simulink model "tumbling_sim_v4"  (R2018a)
settings: Solver=VariableStepAuto  StartTime=0.0  StopTime=10
values from neighbouring files (symbols this model uses):
  q0 = [0.8034 0.1600 0.4272 0.3828]'    [init_tumbling.m]
  qd0 = [0.0379 0.6999 -0.2503 -0.0927]'    [init_tumbling.m]
settings Model: Creator=abinalexpothen  LastModifiedBy=abinalexpothen

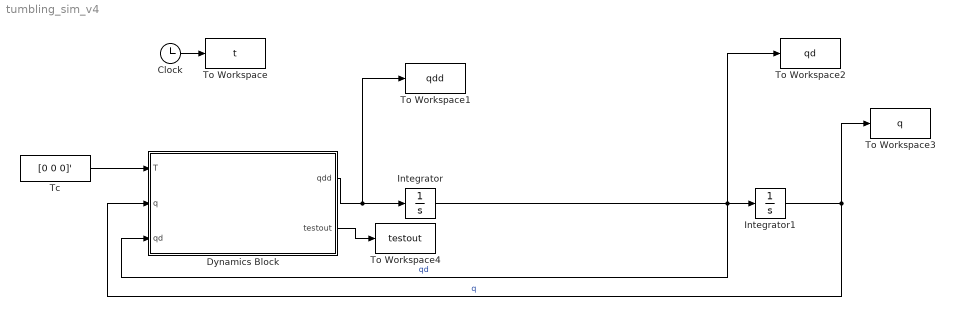
== system tumbling_sim_v4 ==
  Clock : Clock
  Dynamics Block : MATLAB Function  TreatAsAtomicUnit=on
  Integrator : Integrator  InitialCondition=qd0
  Integrator1 : Integrator  InitialCondition=q0
  Tc : Constant  Value=[0 0 0]'
  To Workspace : ToWorkspace  VariableName=t  SampleTime=-1
  To Workspace1 : ToWorkspace  VariableName=qdd  SampleTime=-1
  To Workspace2 : ToWorkspace  VariableName=qd  SampleTime=-1
  To Workspace3 : ToWorkspace  VariableName=q  SampleTime=-1
  To Workspace4 : ToWorkspace  VariableName=testout  SampleTime=-1
  wires:
  Clock/1 -> To Workspace/1
  Dynamics Block/1(qdd) -> To Workspace1/1, Integrator/1
  Integrator/1 -> Dynamics Block/3(qd), To Workspace2/1, Integrator1/1  "qd"
  Integrator1/1 -> To Workspace3/1, Dynamics Block/2(q)  "q"
  Tc/1 -> Dynamics Block/1(T)
  Dynamics Block/2(testout) -> To Workspace4/1

== matlab function tumbling_sim_v4/Dynamics Block ==
  data: T input; qdd output; q input; qd input; J parameter; testout output
function [qdd, testout] = tumbling_dynamics(T, q, qd, J)

H = 2*[-q(2) q(1) q(4) -q(3);
       -q(3) -q(4) q(1) q(2);
       -q(4) q(3) -q(2) q(1)];

qdd = (H'*J*H)\H'*(T-cross(H*qd,J*H*qd))-(q*q')\q*(qd')*qd;
testout = norm(q);
